simulink model "LQG_UAV_LonAP"  (R2019b)
settings: Solver=FixedStepAuto  StartTime=0.0  StopTime=20  FixedStep=0.005  RelTol=1e-3
values from neighbouring files (symbols this model uses):
  Ap = [-0.00403548 0.0511006 0 -3.711; -0.155603 -1.04255 126.189 0; 0.000417069 -3.3536 -1.15905 0; 0 0 1 0 ]    [LonAP_FilghtWing.m]
  Bp = [1.390234 -4.430383 -70.44032 0]'    [LonAP_FilghtWing.m]
  Clo = [0 0 1 0; 0 0 0 1]    [LonAP_FilghtWing.m]
  Cp = eye(4)    [LonAP_FilghtWing.m]
  Dp = zeros(4,1)    [LonAP_FilghtWing.m]
  flag_act = flag_act_aux(i)    [runLQGSimulink.m]
  flag_controller = flag_controller_aux(i)    [runLQGSimulink.m]
  flag_noise = flag_noise_aux(i)    [runLQGSimulink.m]
  Klqg = lqe(Ap,eye(4),Clo, Qf, Rn)    [LonAP_FilghtWing.m]
  Klqr_gain = lqr(A_aug,B_aug, Q , R)    [LonAP_FilghtWing.m]
  wn_act = 5*2*pi    (= 31.4159265359)    [LateralAP_FlightWing.m]    (also in LonAP_FilghtWing.m)
  zeta_act = 0.7    [LateralAP_FlightWing.m]    (also in LonAP_FilghtWing.m)
libraries: simulink x1
settings Model: Creator=adolf  LastModifiedBy=covasanvictor
settings DataIOCC: ReturnWorkspaceOutputs=off
settings DebuggingCC: ArithmeticOperatorsInVariantConditions=warning
settings SFSimCC: SimUseLocalCustomCode=off  CustomCodeUndefinedFunction=UseInterfaceOnly
settings RTWCC: RTWUseLocalCustomCode=off

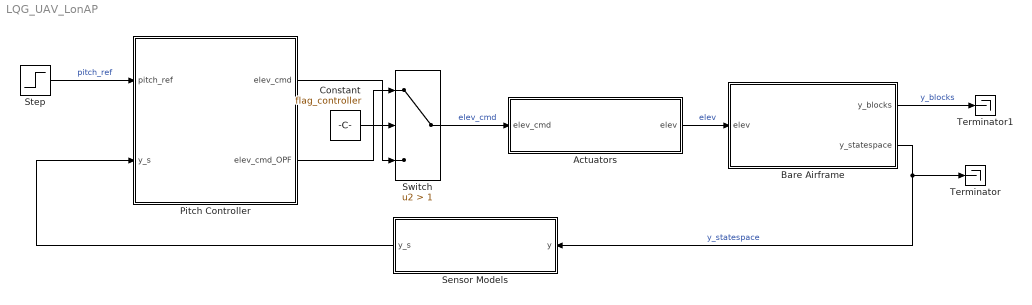
== system LQG_UAV_LonAP ==
  Actuators : Subsystem
  Bare Airframe : Subsystem
  Constant : Constant  Value=flag_controller
  Pitch Controller : Subsystem
  Sensor Models : Subsystem
  Step : Step  SampleTime=0
  Switch : Switch  Criteria=u2 > Threshold  Threshold=1
  Terminator : Terminator
  Terminator1 : Terminator
  wires:
  Bare Airframe/1(y_blocks) -> Terminator1/1  "y_blocks"
  Bare Airframe/2(y_statespace) -> Sensor Models/1(y), Terminator/1  "y_statespace"
  Actuators/1(elev) -> Bare Airframe/1(elev)  "elev"
  Sensor Models/1(y_s) -> Pitch Controller/2("y_s ")
  Step/1 -> Pitch Controller/1(pitch_ref)  "pitch_ref"
  Switch/1 -> Actuators/1(elev_cmd)  "elev_cmd"
  Constant/1 -> Switch/2
  Pitch Controller/2(elev_cmd_OPF) -> Switch/1
  Pitch Controller/1(elev_cmd) -> Switch/3

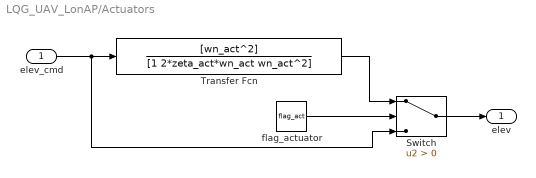
== system LQG_UAV_LonAP/Actuators ==
  elev_cmd : Inport
  Switch : Switch  Criteria=u2 > Threshold
  Transfer Fcn : TransferFcn  Numerator=[wn_act^2]  Denominator=[1 2*zeta_act*wn_act wn_act^2]
  flag_actuator : Constant  Value=flag_act
  elev : Outport  VectorParamsAs1DForOutWhenUnconnected=off
  wires:
  flag_actuator/1 -> Switch/2
  Switch/1 -> elev/1
  Transfer Fcn/1 -> Switch/1
  elev_cmd/1 -> Switch/3, Transfer Fcn/1

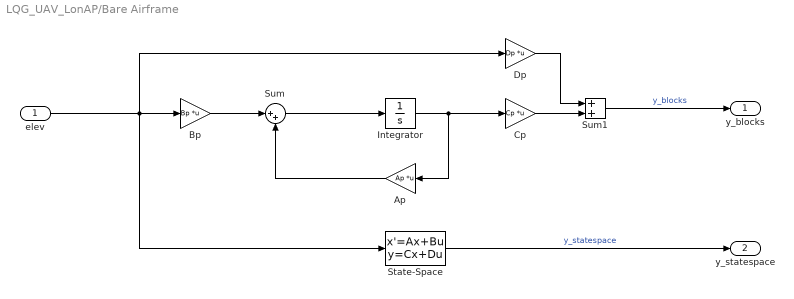
== system LQG_UAV_LonAP/Bare Airframe ==
  elev : Inport
  Ap : Gain  Gain=Ap  Multiplication=Matrix(K*u) (u vector)
  Bp : Gain  Gain=Bp  Multiplication=Matrix(K*u) (u vector)
  Cp : Gain  Gain=Cp  Multiplication=Matrix(K*u) (u vector)
  Dp : Gain  Gain=Dp  Multiplication=Matrix(K*u) (u vector)
  Integrator : Integrator  InitialCondition=zeros(4,1)  ContinuousStateAttributes={'u', 'w','q','theta'}
  State-Space : StateSpace  A=Ap  B=Bp  C=Cp  D=Dp  InitialCondition=0
  Sum : Sum  Inputs=|++
  Sum1 : Sum
  y_blocks : Outport  VectorParamsAs1DForOutWhenUnconnected=off
  y_statespace : Outport  Port=2  VectorParamsAs1DForOutWhenUnconnected=off
  wires:
  State-Space/1 -> y_statespace/1  "y_statespace"
  Cp/1 -> Sum1/2
  Integrator/1 -> Ap/1, Cp/1
  Ap/1 -> Sum/2
  Bp/1 -> Sum/1
  elev/1 -> State-Space/1, Dp/1, Bp/1
  Dp/1 -> Sum1/1
  Sum/1 -> Integrator/1
  Sum1/1 -> y_blocks/1  "y_blocks"

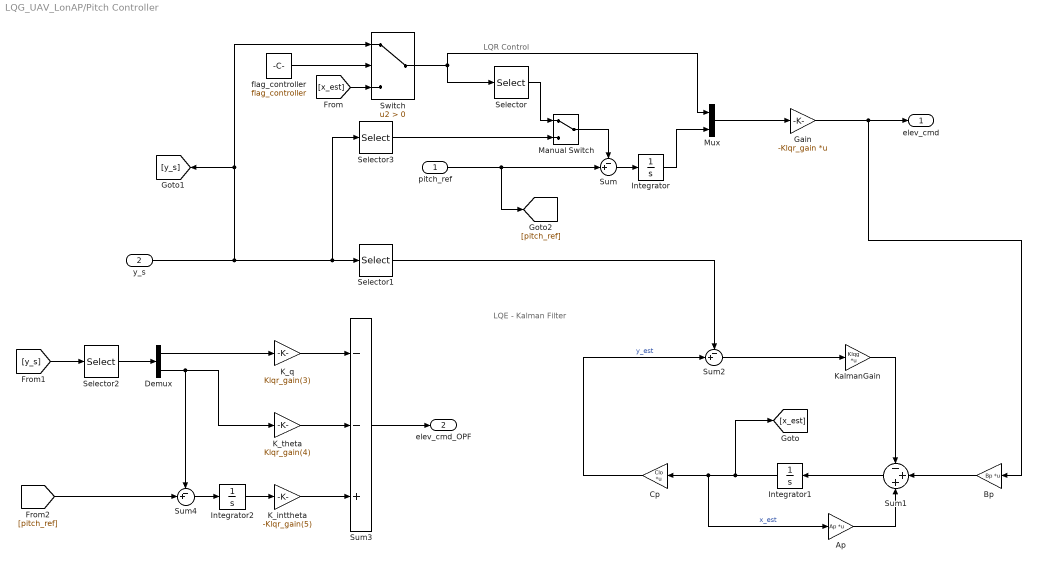
== system LQG_UAV_LonAP/Pitch Controller ==
  note: LQR Control
  note: LQE - Kalman Filter
  pitch_ref : Inport
  "y_s " : Inport  Port=2
  Ap : Gain  Gain=Ap  Multiplication=Matrix(K*u) (u vector)
  Bp : Gain  Gain=Bp  Multiplication=Matrix(K*u) (u vector)
  Cp : Gain  Gain=Clo  Multiplication=Matrix(K*u) (u vector)
  Demux : Demux  Outputs=2
  Gain : Gain  Gain=-Klqr_gain  Multiplication=Matrix(K*u) (u vector)
  Integrator : Integrator
  Integrator1 : Integrator  InitialCondition=zeros(4,1)  ContinuousStateAttributes={'u', 'w','q','theta'}
  Integrator2 : Integrator
  K_inttheta : Gain  Gain=-Klqr_gain(5)
  K_q : Gain  Gain=Klqr_gain(3)
  K_theta : Gain  Gain=Klqr_gain(4)
  KalmanGain : Gain  Gain=Klqg  Multiplication=Matrix(K*u) (u vector)
  Manual Switch : ManualSwitch
  Mux : Mux  Inputs=2
  Selector : Selector  InputPortWidth=4  IndexOptions=Index vector (dialog)  Indices=4  OutputSizes=1
  Selector1 : Selector  InputPortWidth=4  IndexOptions=Index vector (dialog)  Indices=[3 4]  OutputSizes=1
  Selector2 : Selector  InputPortWidth=4  IndexOptions=Index vector (dialog)  Indices=[3 4]  OutputSizes=1
  Selector3 : Selector  InputPortWidth=4  IndexOptions=Index vector (dialog)  Indices=4  OutputSizes=1
  Sum : Sum  Inputs=-+|
  Sum1 : Sum  Inputs=-++
  Sum2 : Sum  Inputs=-+|
  Sum3 : Sum  Inputs=--+
  Sum4 : Sum  Inputs=-+|
  Switch : Switch  Criteria=u2 > Threshold
  flag_controller : Constant  Value=flag_controller
  elev_cmd : Outport  VectorParamsAs1DForOutWhenUnconnected=off
  elev_cmd_OPF : Outport  Port=2  VectorParamsAs1DForOutWhenUnconnected=off
  wires:
  pitch_ref/1 -> [pitch_ref], Sum/2
  Mux/1 -> Gain/1
  Sum/1 -> Integrator/1
  Integrator/1 -> Mux/2
  Gain/1 -> Bp/1, elev_cmd/1
  Sum1/1 -> Integrator1/1
  Integrator1/1 -> [x_est], Cp/1, Ap/1  "x_est"
  Ap/1 -> Sum1/3
  Bp/1 -> Sum1/2
  Cp/1 -> Sum2/2  "y_est"
  Selector1/1 -> Sum2/1
  Sum2/1 -> KalmanGain/1
  Switch/1 -> Selector/1, Mux/1
  flag_controller/1 -> Switch/2
  "y_s "/1 -> Switch/1, [y_s], Selector3/1, Selector1/1
  [x_est] -> Switch/3
  KalmanGain/1 -> Sum1/1
  Sum4/1 -> Integrator2/1
  Integrator2/1 -> K_inttheta/1
  [y_s] -> Selector2/1
  Selector2/1 -> Demux/1
  Demux/1 -> K_q/1
  Demux/2 -> Sum4/1, K_theta/1
  K_q/1 -> Sum3/1
  K_theta/1 -> Sum3/2
  K_inttheta/1 -> Sum3/3
  [pitch_ref] -> Sum4/2
  Sum3/1 -> elev_cmd_OPF/1
  Selector3/1 -> Manual Switch/2
  Manual Switch/1 -> Sum/1
  Selector/1 -> Manual Switch/1

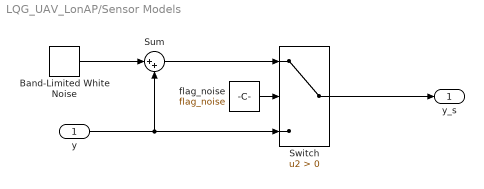
== system LQG_UAV_LonAP/Sensor Models ==
  y : Inport
  Band-Limited White Noise : simulink/Sources/Band-Limited White Noise  Cov=[0.0005 0.0005 0.0005 0.0001]  Ts=0.01  seed=[23341 23342 23343 23344]
  Sum : Sum  Inputs=|++
  Switch : Switch  Criteria=u2 > Threshold
  flag_noise : Constant  Value=flag_noise
  y_s : Outport  VectorParamsAs1DForOutWhenUnconnected=off
  wires:
  flag_noise/1 -> Switch/2
  Switch/1 -> y_s/1
  y/1 -> Sum/2, Switch/3
  Sum/1 -> Switch/1
  Band-Limited White Noise/1 -> Sum/1
